simulink model "LimberoGrieel_Robot_Control"  (R2022a)
settings: Solver=VariableStepAuto  StartTime=0.0  StopTime=10.0  RelTol=1e-3
values from neighbouring files (symbols this model uses):
  a = annotation('textbox',dim,'String',str,'FontSize', 20, 'FitBoxToText','on', 'Interpreter', 'tex')    [Experiment_Plot_csv.m]    (also in GRIEEL_transform.m; Gazebo_Plot_csv.m; Grasshopper_Manipulability.m = [a_1; a_2; a_3]; Hexapod_Manipulability_Develop_limits.m = [0, a2, a3])
  alpha = [alpha; alpha; alpha]    [Grasshopper_Manipulability.m]    (also in Hexapod_Manipulability_Develop_limits.m = [-pi/2, 0, 0]; LimberoGrieel_Leg_DH_Modeling_Control.m = [-pi/2,0,0,-pi/2,pi/2, -pi/2, 0]; NewLimbManipulabilityTest.m = [-pi/2, 0, 0]; NewRobot_Manipulability_Develop.m = [-pi/2, 0, 0])
  d = [d; d; d; d]    [Grasshopper_Manipulability.m]    (also in Hexapod_Manipulability_Develop_limits.m = [0, 0, 0]; LimberoGrieel_Leg_DH_Modeling_Control.m = [0,0,0,0,d5,0,d7]; NewLimbManipulabilityTest.m = [d1, 0, 0]; NewRobot_Manipulability_Develop.m = [0,0,0])
  kpp = w_cp    (= 10)    [LimberoGrieel_Leg_DH_Modeling_Control.m]    (also in limberoGrieel_leg_DH.m = 20; limbero_controller.mat; limbero_grieel_dh.m = 20)
  kpv = zeros(1,7)    [LimberoGrieel_Leg_DH_Modeling_Control.m]    (also in limberoGrieel_leg_DH.m; limbero_controller.mat = [361.812023748 321.153278445 225.192840226 266.564703352 222; limbero_grieel_dh.m)
  masses = zeros(N_link,1)    [LimberoGrieel_Leg_DH_Modeling_Control.m]    (also in limberoGrieel_leg_DH.m; limbero_controller.mat = [0.09109 0.12821 0.061841 0.081999 0.110299813858 0.13265995; limbero_grieel_dh.m)
  offset = [offset; offset; offset]    [Grasshopper_Manipulability.m]    (also in Hexapod_Manipulability_Develop_limits.m = [0, 0, 0]; LimberoGrieel_Leg_DH_Modeling_Control.m = zeros(N_link,1); NewLimbManipulabilityTest.m = [0, 0, 0]; NewRobot_Manipulability_Develop.m = [0, 0, 0])
  q0_contact = {}    [LimberoGrieel_Leg_DH_Modeling_Control.m]    (also in LimberoGrieel_Manipulability_Develop.m = q0; LimberoGrieel_Manipulability_Develop_limits.m = q0_wheel; LimberoGrieel_Manipulability_Develop_mesh.m = q0_wheel; LimberoGrieel_Manipulability_Transform.m = q0_wheel)
  r_cm = zeros(N_link,3)    [LimberoGrieel_Leg_DH_Modeling_Control.m]    (also in limberoGrieel_leg_DH.m; limbero_controller.mat = [-0.015062 -0.09917 -0.09702 -9.53000073933e-12 -0.012686054; limbero_grieel_dh.m)
  ROBOT = Robot_model(W, L, Limb, q0, [1 1 1 1], T_tool)    [Experiment_Plot_csv.m]    (also in Gazebo_Plot_csv.m; Grasshopper_Manipulability.m = Robot_model_general(W, L, Limbs, limbs_place,limbs_angle, q0; Hexapod_Manipulability_Develop_limits.m = Robot_model_general(W, L, Limbs, limbs_place,limbs_angle, q0; LimberoGrieel_Manipulability_Develop.m = Robot_model(W, L, Limb, q0_contact_swing, [1 1 1 1], T_tool))
  T_lpf = 1/(w_lpf*2*pi)    (= 0.0106103295395)    [LimberoGrieel_Leg_DH_Modeling_Control.m]    (also in limberoGrieel_leg_DH.m; limbero_controller.mat; limbero_grieel_dh.m)
  T_vel = 1/(w_vel*2*pi)    (= 0.00318309886184)    [LimberoGrieel_Leg_DH_Modeling_Control.m]    (also in limberoGrieel_leg_DH.m; limbero_controller.mat; limbero_grieel_dh.m)
  Tc = Tiv*0.1    (= 0.0666666666667)    [LimberoGrieel_Leg_DH_Modeling_Control.m]    (also in limberoGrieel_leg_DH.m = 0.0333333333333; limbero_controller.mat; limbero_grieel_dh.m = 0.0333333333333)
  Tiv = Tiv*10    (= 0.666666666667)    [LimberoGrieel_Leg_DH_Modeling_Control.m]    (also in limberoGrieel_leg_DH.m = 0.333333333333; limbero_controller.mat; limbero_grieel_dh.m = 0.333333333333)
libraries: roblocks x12
(part 1 of 2)
settings Model: Creator=ale  LastModifiedBy=ale

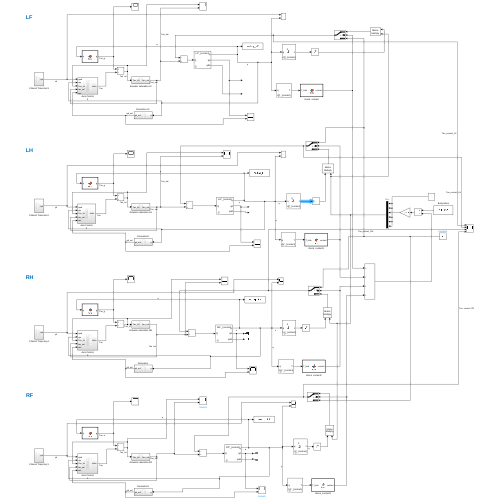
[thumbnail: Simulink's stored preview of the top-level diagram]
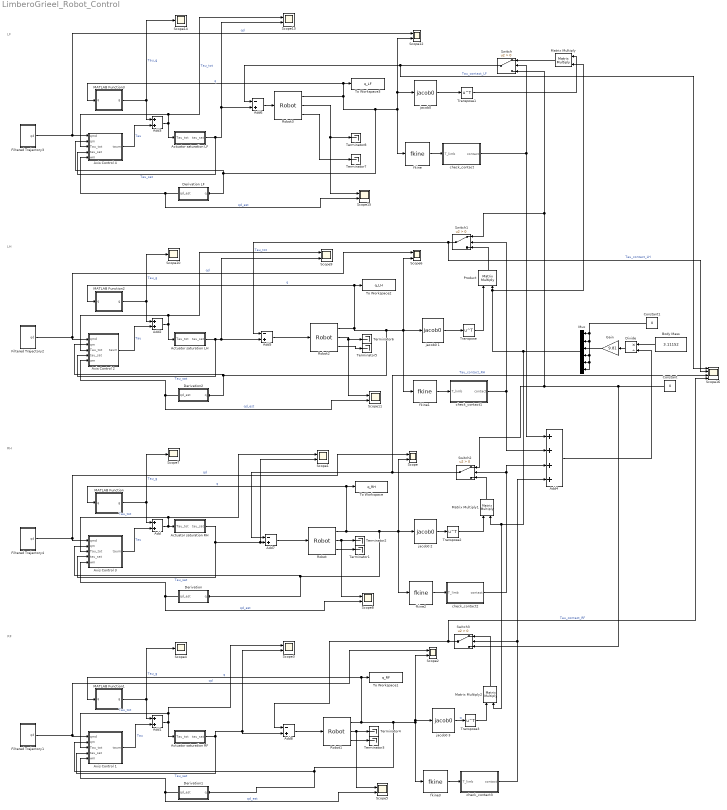
== system LimberoGrieel_Robot_Control ==
  note: RH
  note: RF
  note: LH
  note: LF
  Actuator saturation LF : Subsystem
  Actuator saturation LH : Subsystem
  "Actuator saturation RF " : Subsystem
  Actuator saturation RH : Subsystem
  Add{,1..3} (4 alike) : Sum
  Add4 : Sum  Inputs=++++
  Add{5..8} (4 alike) : Sum  Inputs=-+
  Axis Control 1 : Subsystem
  Axis Control 2 : Subsystem
  Axis Control 3 : Subsystem
  Axis Control 4 : Subsystem
  Body Mass : Constant  Value=3.11152
  Constant : Constant  Value=0
  Constant1 : Constant  Value=0
  Derivation : Subsystem
  Derivation LF : Subsystem
  Derivation1 : Subsystem
  Derivation2 : Subsystem
  Divide : Product  Inputs=*/
  Filtered Trajectory1 : Subsystem
  Filtered Trajectory2 : Subsystem
  Filtered Trajectory3 : Subsystem
  Filtered Trajectory4 : Subsystem
  Gain : Gain  Gain=9.81
  MATLAB Function : MATLAB Function  TreatAsAtomicUnit=on
  MATLAB Function1 : MATLAB Function  TreatAsAtomicUnit=on
  MATLAB Function2 : MATLAB Function  TreatAsAtomicUnit=on
  MATLAB Function3 : MATLAB Function  TreatAsAtomicUnit=on
  Matrix Multiply : Product  Multiplication=Matrix(*)
  Matrix Multiply1 : Product  Multiplication=Matrix(*)
  Matrix Multiply2 : Product  Multiplication=Matrix(*)
  Mux : Mux  Inputs=6
  Product : Product  Multiplication=Matrix(*)
  Robot : roblocks/Arm/Robot  robot=ROBOT(3)  q0=q0_contact(3,:)
  Robot1 : roblocks/Arm/Robot  robot=ROBOT(4)  q0=q0_contact(4,:)
  Robot2 : roblocks/Arm/Robot  robot=ROBOT(2)  q0=q0_contact(2,:)
  Robot3 : roblocks/Arm/Robot  robot=ROBOT(1)  q0=q0_contact(1,:)
  Scope{,1..3,5..6,8..9,11..13,15} (12 alike) : Scope  NumInputPorts=2
  Scope{4,7,10,14} (4 alike) : Scope
  Scope16 : Scope  NumInputPorts=4
  Switch{,1..3} (4 alike) : Switch  Criteria=u2 > Threshold  SaturateOnIntegerOverflow=off  InputSameDT=off
  Terminator{1..8} (8 alike) : Terminator
  To Workspace : ToWorkspace  VariableName=q_RH  SaveFormat=Timeseries  SampleTime=-1
  To Workspace1 : ToWorkspace  VariableName=q_RF  SaveFormat=Timeseries  SampleTime=-1
  To Workspace2 : ToWorkspace  VariableName=q_LH  SaveFormat=Timeseries  SampleTime=-1
  To Workspace3 : ToWorkspace  VariableName=q_LF  SaveFormat=Timeseries  SampleTime=-1
  Transpose{,1..3} (4 alike) : Math  Operator=transpose
  check_contact : MATLAB Function  TreatAsAtomicUnit=on
  check_contact1 : MATLAB Function  TreatAsAtomicUnit=on
  check_contact2 : MATLAB Function  TreatAsAtomicUnit=on
  check_contact3 : MATLAB Function  TreatAsAtomicUnit=on
  fkine : roblocks/Arm/fkine  robot=ROBOT(1)
  fkine1 : roblocks/Arm/fkine  robot=ROBOT(2)
  fkine2 : roblocks/Arm/fkine  robot=ROBOT(3)
  fkine3 : roblocks/Arm/fkine  robot=ROBOT(4)
  "jacob0 " : roblocks/Arm/jacob0   robot=ROBOT(1)
  jacob0 1 : roblocks/Arm/jacob0   robot=ROBOT(2)
  jacob0 2 : roblocks/Arm/jacob0   robot=ROBOT(3)
  jacob0 3 : roblocks/Arm/jacob0   robot=ROBOT(4)
  wires:
  Axis Control 3/1("taum ") -> Add/2  "Tau"
  Robot/3 -> Terminator1/1
  MATLAB Function/1(g) -> Add/1, Scope7/1  "Tau_g"
  Actuator saturation RH/1(tau_sat) -> Scope1/2, Add7/2, Axis Control 3/4(tau_sat)  "Tau_sat"
  Derivation/1(qd_est) -> Scope8/2, Axis Control 3/5(wm)  "qd_est"
  Add/1 -> Axis Control 3/3(Tau_tot), Scope1/1, Actuator saturation RH/1(Tau_tot)  "Tau_tot"
  Filtered Trajectory4/1(qd) -> Axis Control 3/1(qmd), Scope/1  "qd"
  Robot/2 -> Scope8/1, Terminator2/1
  Axis Control 1/1("taum ") -> Add1/2  "Tau"
  Robot1/3 -> Terminator3/1
  MATLAB Function1/1(g) -> Add1/1, Scope4/1  "Tau_g"
  "Actuator saturation RF "/1(tau_sat) -> Axis Control 1/4(tau_sat), Add8/2, Scope3/2  "Tau_sat"
  Derivation1/1(qd_est) -> Scope5/2, Axis Control 1/5(wm)  "qd_est"
  Add1/1 -> Axis Control 1/3(Tau_tot), Scope3/1, "Actuator saturation RF "/1(Tau_tot)  "Tau_tot"
  Filtered Trajectory1/1(qd) -> Axis Control 1/1(qmd), Scope2/1  "qd"
  Robot1/2 -> Scope5/1, Terminator4/1
  Axis Control 2/1("taum ") -> Add2/2  "Tau"
  Robot2/3 -> Terminator5/1
  MATLAB Function2/1(g) -> Add2/1, Scope10/1  "Tau_g"
  Actuator saturation LH/1(tau_sat) -> Axis Control 2/4(tau_sat), Add5/2, Scope9/2  "Tau_sat"
  Derivation2/1(qd_est) -> Scope11/2, Axis Control 2/5(wm)  "qd_est"
  Add2/1 -> Axis Control 2/3(Tau_tot), Scope9/1, Actuator saturation LH/1(Tau_tot)  "Tau_tot"
  Filtered Trajectory2/1(qd) -> Axis Control 2/1(qmd), Scope6/1  "qd"
  Robot2/2 -> Scope11/1, Terminator6/1
  Robot3/1 -> Derivation LF/1(q), Axis Control 4/2(qm), fkine/1, Scope12/2, "jacob0 "/1, MATLAB Function3/1(q), To Workspace3/1  "q"
  Axis Control 4/1("taum ") -> Add3/2  "Tau"
  Robot3/3 -> Terminator7/1
  MATLAB Function3/1(g) -> Add3/1, Scope14/1  "Tau_g"
  Actuator saturation LF/1(tau_sat) -> Axis Control 4/4(tau_sat), Add6/2, Scope13/2  "Tau_sat"
  Derivation LF/1(qd_est) -> Scope15/2, Axis Control 4/5(wm)  "qd_est"
  Add3/1 -> Axis Control 4/3(Tau_tot), Scope13/1, Actuator saturation LF/1(Tau_tot)  "Tau_tot"
  Filtered Trajectory3/1(qd) -> Axis Control 4/1(qmd), Scope12/1  "qd"
  Robot3/2 -> Terminator8/1, Scope15/1
  fkine/1 -> check_contact/1(T_limb)
  Add6/1 -> Robot3/1
  check_contact/1(contact) -> Add4/1, Switch/2
  Robot2/1 -> Derivation2/1(q), Axis Control 2/2(qm), fkine1/1, jacob0 1/1, Scope6/2, MATLAB Function2/1(q), To Workspace2/1  "q"
  check_contact1/1(contact) -> Add4/2, Switch1/2
  fkine1/1 -> check_contact1/1(T_limb)
  Robot/1 -> MATLAB Function/1(q), To Workspace/1, Derivation/1(q), Axis Control 3/2(qm), fkine2/1, jacob0 2/1, Scope/2  "q"
  check_contact2/1(contact) -> Add4/3, Switch2/2
  fkine2/1 -> check_contact2/1(T_limb)
  Robot1/1 -> MATLAB Function1/1(q), To Workspace1/1, Axis Control 1/2(qm), Derivation1/1(q), jacob0 3/1, Scope2/2, fkine3/1  "q"
  check_contact3/1(contact) -> Add4/4, Switch3/2
  fkine3/1 -> check_contact3/1(T_limb)
  Body Mass/1 -> Divide/1
  Add4/1 -> Divide/2
  Divide/1 -> Gain/1
  jacob0 1/1 -> Transpose/1
  Gain/1 -> Mux/3
  Product/1 -> Switch1/3
  Constant/1 -> Switch3/3, Switch1/1, Switch/3, Switch2/1
  Add5/1 -> Robot2/1
  Switch1/1 -> Add5/1, Scope16/2  "Tau_contact_LH"
  Transpose/1 -> Product/1
  "jacob0 "/1 -> Transpose1/1
  Transpose1/1 -> Matrix Multiply/1
  Matrix Multiply/1 -> Switch/1
  Switch/1 -> Scope16/1, Add6/1  "Tau_contact_LF"
  jacob0 2/1 -> Transpose2/1
  Transpose2/1 -> Matrix Multiply1/1
  Matrix Multiply1/1 -> Switch2/3
  Add7/1 -> Robot/1
  Switch2/1 -> Add7/1, Scope16/3  "Tau_contact_RH"
  jacob0 3/1 -> Transpose3/1  "q"
  Transpose3/1 -> Matrix Multiply2/1
  Matrix Multiply2/1 -> Switch3/1
  Add8/1 -> Robot1/1
  Switch3/1 -> Scope16/4, Add8/1  "Tau_contact_RF"
  Constant1/1 -> Mux/6, Mux/5, Mux/4, Mux/2, Mux/1
  Mux/1 -> Matrix Multiply1/2, Matrix Multiply2/2, Matrix Multiply/2, Product/2

== system LimberoGrieel_Robot_Control/Actuator saturation LF ==
  Tau_tot : Inport
  Demux : Demux  Outputs=7
  Mux : Mux  Inputs=7
  Saturation : Saturate  UpperLimit=20.0  LowerLimit=-20.0
  Saturation1 : Saturate  UpperLimit=20.0  LowerLimit=-20.0
  Saturation2 : Saturate  UpperLimit=12.0  LowerLimit=-12.0
  Saturation3 : Saturate  UpperLimit=14.0  LowerLimit=-14.0
  Saturation4 : Saturate  UpperLimit=12.0  LowerLimit=-12.0
  Saturation5 : Saturate  UpperLimit=14.0  LowerLimit=-14.0
  Saturation6 : Saturate  UpperLimit=12.0  LowerLimit=-12.0
  tau_sat : Outport
  wires:
  Saturation6/1 -> Mux/7
  Mux/1 -> tau_sat/1
  Saturation3/1 -> Mux/4
  Tau_tot/1 -> Demux/1
  Demux/4 -> Saturation3/1
  Demux/7 -> Saturation6/1
  Saturation4/1 -> Mux/5
  Saturation1/1 -> Mux/2
  Demux/3 -> Saturation2/1
  Demux/1 -> Saturation/1
  Demux/5 -> Saturation4/1
  Demux/6 -> Saturation5/1
  Demux/2 -> Saturation1/1
  Saturation/1 -> Mux/1
  Saturation5/1 -> Mux/6
  Saturation2/1 -> Mux/3

== system LimberoGrieel_Robot_Control/Actuator saturation LH ==
  Tau_tot : Inport
  Demux : Demux  Outputs=7
  Mux : Mux  Inputs=7
  Saturation : Saturate  UpperLimit=20.0  LowerLimit=-20.0
  Saturation1 : Saturate  UpperLimit=20.0  LowerLimit=-20.0
  Saturation2 : Saturate  UpperLimit=12.0  LowerLimit=-12.0
  Saturation3 : Saturate  UpperLimit=14.0  LowerLimit=-14.0
  Saturation4 : Saturate  UpperLimit=12.0  LowerLimit=-12.0
  Saturation5 : Saturate  UpperLimit=14.0  LowerLimit=-14.0
  Saturation6 : Saturate  UpperLimit=12.0  LowerLimit=-12.0
  tau_sat : Outport
  wires:
  Saturation6/1 -> Mux/7
  Mux/1 -> tau_sat/1
  Saturation3/1 -> Mux/4
  Tau_tot/1 -> Demux/1
  Demux/4 -> Saturation3/1
  Demux/7 -> Saturation6/1
  Saturation4/1 -> Mux/5
  Saturation1/1 -> Mux/2
  Demux/3 -> Saturation2/1
  Demux/1 -> Saturation/1
  Demux/5 -> Saturation4/1
  Demux/6 -> Saturation5/1
  Demux/2 -> Saturation1/1
  Saturation/1 -> Mux/1
  Saturation5/1 -> Mux/6
  Saturation2/1 -> Mux/3

== system LimberoGrieel_Robot_Control/Actuator saturation RF  ==
  Tau_tot : Inport
  Demux : Demux  Outputs=7
  Mux : Mux  Inputs=7
  Saturation : Saturate  UpperLimit=20.0  LowerLimit=-20.0
  Saturation1 : Saturate  UpperLimit=20.0  LowerLimit=-20.0
  Saturation2 : Saturate  UpperLimit=12.0  LowerLimit=-12.0
  Saturation3 : Saturate  UpperLimit=14.0  LowerLimit=-14.0
  Saturation4 : Saturate  UpperLimit=12.0  LowerLimit=-12.0
  Saturation5 : Saturate  UpperLimit=14.0  LowerLimit=-14.0
  Saturation6 : Saturate  UpperLimit=12.0  LowerLimit=-12.0
  tau_sat : Outport
  wires:
  Saturation6/1 -> Mux/7
  Mux/1 -> tau_sat/1
  Saturation3/1 -> Mux/4
  Tau_tot/1 -> Demux/1
  Demux/4 -> Saturation3/1
  Demux/7 -> Saturation6/1
  Saturation4/1 -> Mux/5
  Saturation1/1 -> Mux/2
  Demux/3 -> Saturation2/1
  Demux/1 -> Saturation/1
  Demux/5 -> Saturation4/1
  Demux/6 -> Saturation5/1
  Demux/2 -> Saturation1/1
  Saturation/1 -> Mux/1
  Saturation5/1 -> Mux/6
  Saturation2/1 -> Mux/3

== system LimberoGrieel_Robot_Control/Actuator saturation RH ==
  Tau_tot : Inport
  Demux : Demux  Outputs=7
  Mux : Mux  Inputs=7
  Saturation : Saturate  UpperLimit=20.0  LowerLimit=-20.0
  Saturation1 : Saturate  UpperLimit=20.0  LowerLimit=-20.0
  Saturation2 : Saturate  UpperLimit=12.0  LowerLimit=-12.0
  Saturation3 : Saturate  UpperLimit=14.0  LowerLimit=-14.0
  Saturation4 : Saturate  UpperLimit=12.0  LowerLimit=-12.0
  Saturation5 : Saturate  UpperLimit=14.0  LowerLimit=-14.0
  Saturation6 : Saturate  UpperLimit=12.0  LowerLimit=-12.0
  tau_sat : Outport
  wires:
  Saturation6/1 -> Mux/7
  Mux/1 -> tau_sat/1
  Saturation3/1 -> Mux/4
  Tau_tot/1 -> Demux/1
  Demux/4 -> Saturation3/1
  Demux/7 -> Saturation6/1
  Saturation4/1 -> Mux/5
  Saturation1/1 -> Mux/2
  Demux/3 -> Saturation2/1
  Demux/1 -> Saturation/1
  Demux/5 -> Saturation4/1
  Demux/6 -> Saturation5/1
  Demux/2 -> Saturation1/1
  Saturation/1 -> Mux/1
  Saturation5/1 -> Mux/6
  Saturation2/1 -> Mux/3

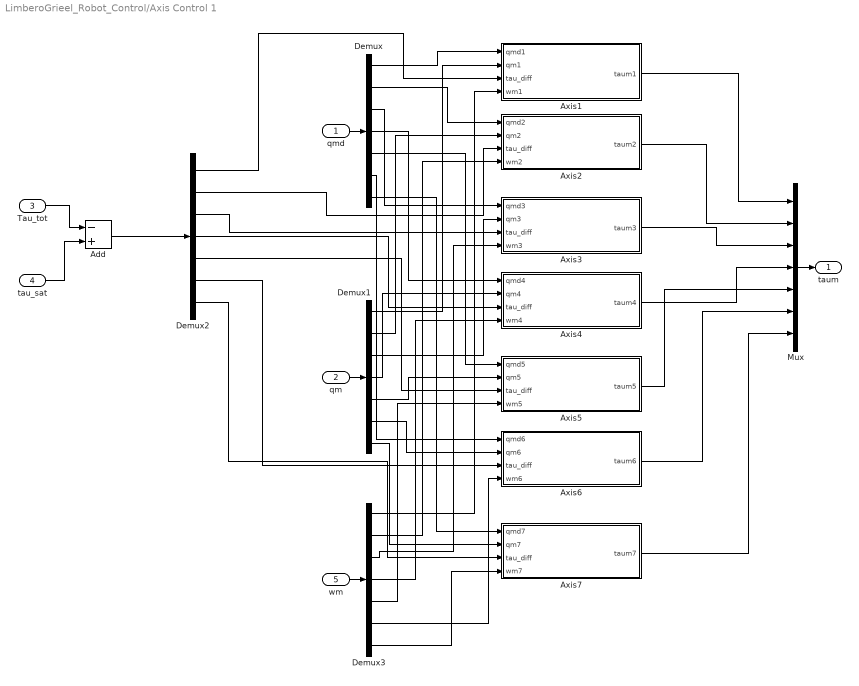
== system LimberoGrieel_Robot_Control/Axis Control 1 ==
  qmd : Inport
  qm : Inport  Port=2
  Tau_tot : Inport  Port=3
  tau_sat : Inport  Port=4
  wm : Inport  Port=5
  Add : Sum  Inputs=-+
  "Axis1 " : Subsystem
  "Axis2 " : Subsystem
  "Axis3 " : Subsystem
  "Axis4 " : Subsystem
  "Axis5 " : Subsystem
  "Axis6 " : Subsystem
  "Axis7 " : Subsystem
  Demux{,1..3} (4 alike) : Demux  Outputs=7
  Mux : Mux  Inputs=7
  "taum " : Outport  VectorParamsAs1DForOutWhenUnconnected=off
  wires:
  "Axis5 "/1(taum5) -> Mux/5
  Demux1/1 -> "Axis1 "/2(qm1)
  "Axis2 "/1(taum2) -> Mux/2
  Demux1/3 -> "Axis3 "/2(qm3)
  Demux/1 -> "Axis1 "/1(qmd1)
  "Axis4 "/1(taum4) -> Mux/4
  "Axis3 "/1(taum3) -> Mux/3
  "Axis6 "/1(taum6) -> Mux/6
  "Axis1 "/1(taum1) -> Mux/1
  Mux/1 -> "taum "/1
  Demux/2 -> "Axis2 "/1(qmd2)
  Demux/4 -> "Axis4 "/1(qmd4)
  Demux/3 -> "Axis3 "/1(qmd3)
  Demux/6 -> "Axis6 "/1(qmd6)
  Demux/5 -> "Axis5 "/1(qmd5)
  Demux1/4 -> "Axis4 "/2(qm4)
  Demux1/6 -> "Axis6 "/2(qm6)
  Demux1/5 -> "Axis5 "/2(qm5)
  Demux1/2 -> "Axis2 "/2(qm2)
  qm/1 -> Demux1/1
  qmd/1 -> Demux/1
  Demux1/7 -> "Axis7 "/2(qm7)
  Demux/7 -> "Axis7 "/1(qmd7)
  "Axis7 "/1(taum7) -> Mux/7
  Tau_tot/1 -> Add/1
  tau_sat/1 -> Add/2
  Demux2/7 -> "Axis7 "/3(tau_diff)
  Add/1 -> Demux2/1
  Demux2/6 -> "Axis6 "/3(tau_diff)
  Demux2/5 -> "Axis5 "/3(tau_diff)
  Demux2/4 -> "Axis4 "/3(tau_diff)
  Demux2/3 -> "Axis3 "/3(tau_diff)
  Demux2/2 -> "Axis2 "/3(tau_diff)
  Demux2/1 -> "Axis1 "/3(tau_diff)
  wm/1 -> Demux3/1
  Demux3/1 -> "Axis1 "/4(wm1)
  Demux3/2 -> "Axis2 "/4(wm2)
  Demux3/3 -> "Axis3 "/4(wm3)
  Demux3/4 -> "Axis4 "/4(wm4)
  Demux3/5 -> "Axis5 "/4(wm5)
  Demux3/6 -> "Axis6 "/4(wm6)
  Demux3/7 -> "Axis7 "/4(wm7)

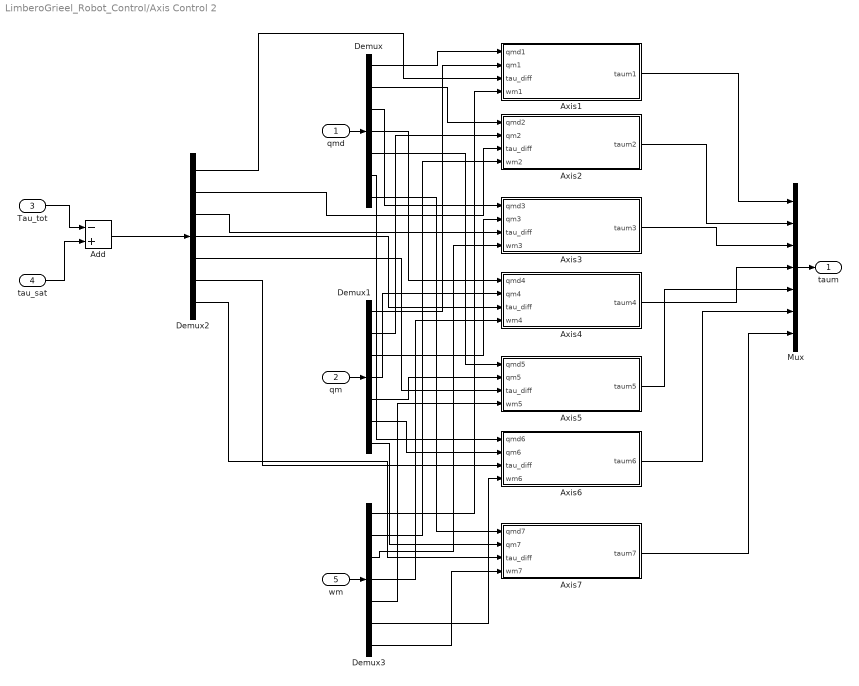
== system LimberoGrieel_Robot_Control/Axis Control 2 ==
  qmd : Inport
  qm : Inport  Port=2
  Tau_tot : Inport  Port=3
  tau_sat : Inport  Port=4
  wm : Inport  Port=5
  Add : Sum  Inputs=-+
  "Axis1 " : Subsystem
  "Axis2 " : Subsystem
  "Axis3 " : Subsystem
  "Axis4 " : Subsystem
  "Axis5 " : Subsystem
  "Axis6 " : Subsystem
  "Axis7 " : Subsystem
  Demux{,1..3} (4 alike) : Demux  Outputs=7
  Mux : Mux  Inputs=7
  "taum " : Outport  VectorParamsAs1DForOutWhenUnconnected=off
  wires:
  "Axis5 "/1(taum5) -> Mux/5
  Demux1/1 -> "Axis1 "/2(qm1)
  "Axis2 "/1(taum2) -> Mux/2
  Demux1/3 -> "Axis3 "/2(qm3)
  Demux/1 -> "Axis1 "/1(qmd1)
  "Axis4 "/1(taum4) -> Mux/4
  "Axis3 "/1(taum3) -> Mux/3
  "Axis6 "/1(taum6) -> Mux/6
  "Axis1 "/1(taum1) -> Mux/1
  Mux/1 -> "taum "/1
  Demux/2 -> "Axis2 "/1(qmd2)
  Demux/4 -> "Axis4 "/1(qmd4)
  Demux/3 -> "Axis3 "/1(qmd3)
  Demux/6 -> "Axis6 "/1(qmd6)
  Demux/5 -> "Axis5 "/1(qmd5)
  Demux1/4 -> "Axis4 "/2(qm4)
  Demux1/6 -> "Axis6 "/2(qm6)
  Demux1/5 -> "Axis5 "/2(qm5)
  Demux1/2 -> "Axis2 "/2(qm2)
  qm/1 -> Demux1/1
  qmd/1 -> Demux/1
  Demux1/7 -> "Axis7 "/2(qm7)
  Demux/7 -> "Axis7 "/1(qmd7)
  "Axis7 "/1(taum7) -> Mux/7
  Tau_tot/1 -> Add/1
  tau_sat/1 -> Add/2
  Demux2/7 -> "Axis7 "/3(tau_diff)
  Add/1 -> Demux2/1
  Demux2/6 -> "Axis6 "/3(tau_diff)
  Demux2/5 -> "Axis5 "/3(tau_diff)
  Demux2/4 -> "Axis4 "/3(tau_diff)
  Demux2/3 -> "Axis3 "/3(tau_diff)
  Demux2/2 -> "Axis2 "/3(tau_diff)
  Demux2/1 -> "Axis1 "/3(tau_diff)
  wm/1 -> Demux3/1
  Demux3/1 -> "Axis1 "/4(wm1)
  Demux3/2 -> "Axis2 "/4(wm2)
  Demux3/3 -> "Axis3 "/4(wm3)
  Demux3/4 -> "Axis4 "/4(wm4)
  Demux3/5 -> "Axis5 "/4(wm5)
  Demux3/6 -> "Axis6 "/4(wm6)
  Demux3/7 -> "Axis7 "/4(wm7)

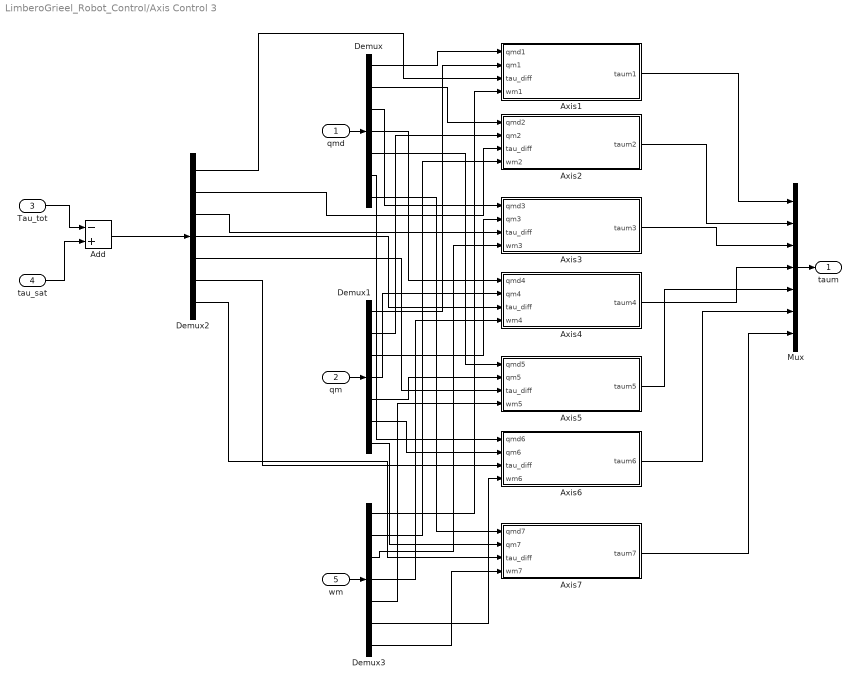
== system LimberoGrieel_Robot_Control/Axis Control 3 ==
  qmd : Inport
  qm : Inport  Port=2
  Tau_tot : Inport  Port=3
  tau_sat : Inport  Port=4
  wm : Inport  Port=5
  Add : Sum  Inputs=-+
  "Axis1 " : Subsystem
  "Axis2 " : Subsystem
  "Axis3 " : Subsystem
  "Axis4 " : Subsystem
  "Axis5 " : Subsystem
  "Axis6 " : Subsystem
  "Axis7 " : Subsystem
  Demux{,1..3} (4 alike) : Demux  Outputs=7
  Mux : Mux  Inputs=7
  "taum " : Outport  VectorParamsAs1DForOutWhenUnconnected=off
  wires:
  "Axis5 "/1(taum5) -> Mux/5
  Demux1/1 -> "Axis1 "/2(qm1)
  "Axis2 "/1(taum2) -> Mux/2
  Demux1/3 -> "Axis3 "/2(qm3)
  Demux/1 -> "Axis1 "/1(qmd1)
  "Axis4 "/1(taum4) -> Mux/4
  "Axis3 "/1(taum3) -> Mux/3
  "Axis6 "/1(taum6) -> Mux/6
  "Axis1 "/1(taum1) -> Mux/1
  Mux/1 -> "taum "/1
  Demux/2 -> "Axis2 "/1(qmd2)
  Demux/4 -> "Axis4 "/1(qmd4)
  Demux/3 -> "Axis3 "/1(qmd3)
  Demux/6 -> "Axis6 "/1(qmd6)
  Demux/5 -> "Axis5 "/1(qmd5)
  Demux1/4 -> "Axis4 "/2(qm4)
  Demux1/6 -> "Axis6 "/2(qm6)
  Demux1/5 -> "Axis5 "/2(qm5)
  Demux1/2 -> "Axis2 "/2(qm2)
  qm/1 -> Demux1/1
  qmd/1 -> Demux/1
  Demux1/7 -> "Axis7 "/2(qm7)
  Demux/7 -> "Axis7 "/1(qmd7)
  "Axis7 "/1(taum7) -> Mux/7
  Tau_tot/1 -> Add/1
  tau_sat/1 -> Add/2
  Demux2/7 -> "Axis7 "/3(tau_diff)
  Add/1 -> Demux2/1
  Demux2/6 -> "Axis6 "/3(tau_diff)
  Demux2/5 -> "Axis5 "/3(tau_diff)
  Demux2/4 -> "Axis4 "/3(tau_diff)
  Demux2/3 -> "Axis3 "/3(tau_diff)
  Demux2/2 -> "Axis2 "/3(tau_diff)
  Demux2/1 -> "Axis1 "/3(tau_diff)
  wm/1 -> Demux3/1
  Demux3/1 -> "Axis1 "/4(wm1)
  Demux3/2 -> "Axis2 "/4(wm2)
  Demux3/3 -> "Axis3 "/4(wm3)
  Demux3/4 -> "Axis4 "/4(wm4)
  Demux3/5 -> "Axis5 "/4(wm5)
  Demux3/6 -> "Axis6 "/4(wm6)
  Demux3/7 -> "Axis7 "/4(wm7)

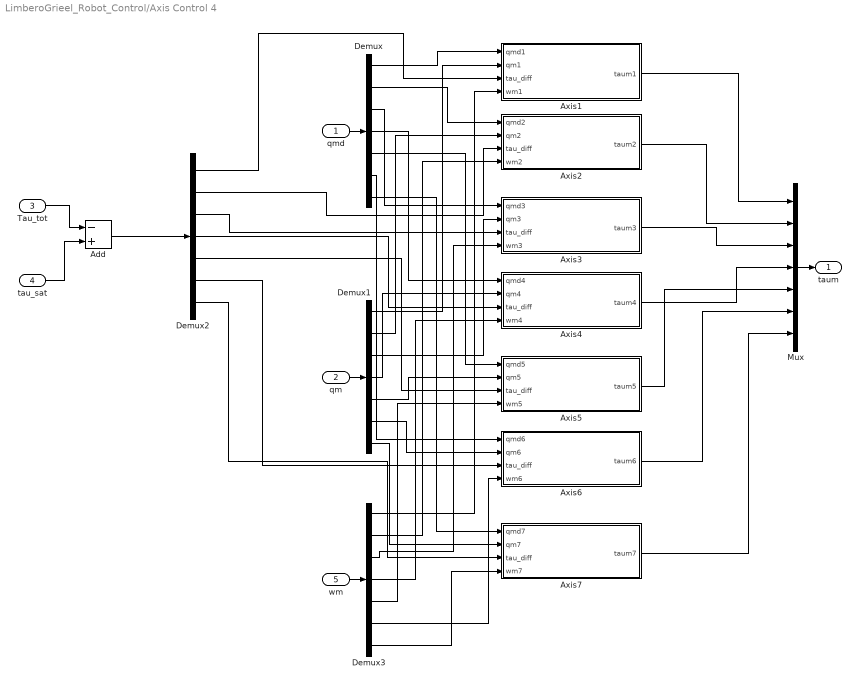
== system LimberoGrieel_Robot_Control/Axis Control 4 ==
  qmd : Inport
  qm : Inport  Port=2
  Tau_tot : Inport  Port=3
  tau_sat : Inport  Port=4
  wm : Inport  Port=5
  Add : Sum  Inputs=-+
  "Axis1 " : Subsystem
  "Axis2 " : Subsystem
  "Axis3 " : Subsystem
  "Axis4 " : Subsystem
  "Axis5 " : Subsystem
  "Axis6 " : Subsystem
  "Axis7 " : Subsystem
  Demux{,1..3} (4 alike) : Demux  Outputs=7
  Mux : Mux  Inputs=7
  "taum " : Outport  VectorParamsAs1DForOutWhenUnconnected=off
  wires:
  "Axis5 "/1(taum5) -> Mux/5
  Demux1/1 -> "Axis1 "/2(qm1)
  "Axis2 "/1(taum2) -> Mux/2
  Demux1/3 -> "Axis3 "/2(qm3)
  Demux/1 -> "Axis1 "/1(qmd1)
  "Axis4 "/1(taum4) -> Mux/4
  "Axis3 "/1(taum3) -> Mux/3
  "Axis6 "/1(taum6) -> Mux/6
  "Axis1 "/1(taum1) -> Mux/1
  Mux/1 -> "taum "/1
  Demux/2 -> "Axis2 "/1(qmd2)
  Demux/4 -> "Axis4 "/1(qmd4)
  Demux/3 -> "Axis3 "/1(qmd3)
  Demux/6 -> "Axis6 "/1(qmd6)
  Demux/5 -> "Axis5 "/1(qmd5)
  Demux1/4 -> "Axis4 "/2(qm4)
  Demux1/6 -> "Axis6 "/2(qm6)
  Demux1/5 -> "Axis5 "/2(qm5)
  Demux1/2 -> "Axis2 "/2(qm2)
  qm/1 -> Demux1/1
  qmd/1 -> Demux/1
  Demux1/7 -> "Axis7 "/2(qm7)
  Demux/7 -> "Axis7 "/1(qmd7)
  "Axis7 "/1(taum7) -> Mux/7
  Tau_tot/1 -> Add/1
  tau_sat/1 -> Add/2
  Demux2/7 -> "Axis7 "/3(tau_diff)
  Add/1 -> Demux2/1
  Demux2/6 -> "Axis6 "/3(tau_diff)
  Demux2/5 -> "Axis5 "/3(tau_diff)
  Demux2/4 -> "Axis4 "/3(tau_diff)
  Demux2/3 -> "Axis3 "/3(tau_diff)
  Demux2/2 -> "Axis2 "/3(tau_diff)
  Demux2/1 -> "Axis1 "/3(tau_diff)
  wm/1 -> Demux3/1
  Demux3/1 -> "Axis1 "/4(wm1)
  Demux3/2 -> "Axis2 "/4(wm2)
  Demux3/3 -> "Axis3 "/4(wm3)
  Demux3/4 -> "Axis4 "/4(wm4)
  Demux3/5 -> "Axis5 "/4(wm5)
  Demux3/6 -> "Axis6 "/4(wm6)
  Demux3/7 -> "Axis7 "/4(wm7)

== system LimberoGrieel_Robot_Control/Derivation ==
  q : Inport
  Demux : Demux  Outputs=7
  Mux : Mux  Inputs=7
  Transfer Fcn{,1..6} (7 alike) : TransferFcn  Numerator=[1 0]  Denominator=[T_vel 1]
  qd_est : Outport
  wires:
  Mux/1 -> qd_est/1
  q/1 -> Demux/1
  Demux/4 -> Transfer Fcn3/1
  Demux/7 -> Transfer Fcn6/1
  Transfer Fcn1/1 -> Mux/2
  Demux/3 -> Transfer Fcn2/1
  Demux/1 -> Transfer Fcn/1
  Demux/5 -> Transfer Fcn4/1
  Demux/6 -> Transfer Fcn5/1
  Demux/2 -> Transfer Fcn1/1
  Transfer Fcn/1 -> Mux/1
  Transfer Fcn6/1 -> Mux/7
  Transfer Fcn5/1 -> Mux/6
  Transfer Fcn4/1 -> Mux/5
  Transfer Fcn3/1 -> Mux/4
  Transfer Fcn2/1 -> Mux/3

== system LimberoGrieel_Robot_Control/Derivation LF ==
  q : Inport
  Demux : Demux  Outputs=7
  Mux : Mux  Inputs=7
  Transfer Fcn{,1..6} (7 alike) : TransferFcn  Numerator=[1 0]  Denominator=[T_vel 1]
  qd_est : Outport
  wires:
  Mux/1 -> qd_est/1
  q/1 -> Demux/1
  Demux/4 -> Transfer Fcn3/1
  Demux/7 -> Transfer Fcn6/1
  Transfer Fcn1/1 -> Mux/2
  Demux/3 -> Transfer Fcn2/1
  Demux/1 -> Transfer Fcn/1
  Demux/5 -> Transfer Fcn4/1
  Demux/6 -> Transfer Fcn5/1
  Demux/2 -> Transfer Fcn1/1
  Transfer Fcn/1 -> Mux/1
  Transfer Fcn6/1 -> Mux/7
  Transfer Fcn5/1 -> Mux/6
  Transfer Fcn4/1 -> Mux/5
  Transfer Fcn3/1 -> Mux/4
  Transfer Fcn2/1 -> Mux/3

== system LimberoGrieel_Robot_Control/Derivation1 ==
  q : Inport
  Demux : Demux  Outputs=7
  Mux : Mux  Inputs=7
  Transfer Fcn{,1..6} (7 alike) : TransferFcn  Numerator=[1 0]  Denominator=[T_vel 1]
  qd_est : Outport
  wires:
  Mux/1 -> qd_est/1
  q/1 -> Demux/1
  Demux/4 -> Transfer Fcn3/1
  Demux/7 -> Transfer Fcn6/1
  Transfer Fcn1/1 -> Mux/2
  Demux/3 -> Transfer Fcn2/1
  Demux/1 -> Transfer Fcn/1
  Demux/5 -> Transfer Fcn4/1
  Demux/6 -> Transfer Fcn5/1
  Demux/2 -> Transfer Fcn1/1
  Transfer Fcn/1 -> Mux/1
  Transfer Fcn6/1 -> Mux/7
  Transfer Fcn5/1 -> Mux/6
  Transfer Fcn4/1 -> Mux/5
  Transfer Fcn3/1 -> Mux/4
  Transfer Fcn2/1 -> Mux/3

== system LimberoGrieel_Robot_Control/Derivation2 ==
  q : Inport
  Demux : Demux  Outputs=7
  Mux : Mux  Inputs=7
  Transfer Fcn{,1..6} (7 alike) : TransferFcn  Numerator=[1 0]  Denominator=[T_vel 1]
  qd_est : Outport
  wires:
  Mux/1 -> qd_est/1
  q/1 -> Demux/1
  Demux/4 -> Transfer Fcn3/1
  Demux/7 -> Transfer Fcn6/1
  Transfer Fcn1/1 -> Mux/2
  Demux/3 -> Transfer Fcn2/1
  Demux/1 -> Transfer Fcn/1
  Demux/5 -> Transfer Fcn4/1
  Demux/6 -> Transfer Fcn5/1
  Demux/2 -> Transfer Fcn1/1
  Transfer Fcn/1 -> Mux/1
  Transfer Fcn6/1 -> Mux/7
  Transfer Fcn5/1 -> Mux/6
  Transfer Fcn4/1 -> Mux/5
  Transfer Fcn3/1 -> Mux/4
  Transfer Fcn2/1 -> Mux/3

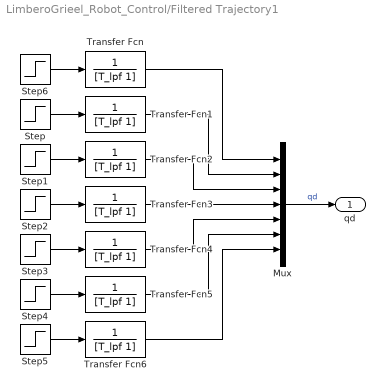
== system LimberoGrieel_Robot_Control/Filtered Trajectory1 ==
  Mux : Mux  Inputs=7
  Step : Step  After=0  SampleTime=0
  Step1 : Step  After=0  SampleTime=0
  Step{2..5} (4 alike) : Step  Time=0  After=0  SampleTime=0
  Step6 : Step  Time=0.5  After=0  SampleTime=0
  Transfer Fcn{,1..6} (7 alike) : TransferFcn  Denominator=[T_lpf 1]
  qd : Outport
  wires:
  Step5/1 -> Transfer Fcn6/1
  Mux/1 -> qd/1  "qd"
  Transfer Fcn1/1 -> Mux/2
  Transfer Fcn4/1 -> Mux/5
  Transfer Fcn2/1 -> Mux/3
  Step6/1 -> Transfer Fcn/1
  Step/1 -> Transfer Fcn1/1
  Step2/1 -> Transfer Fcn3/1
  Transfer Fcn5/1 -> Mux/6
  Transfer Fcn3/1 -> Mux/4
  Transfer Fcn6/1 -> Mux/7
  Transfer Fcn/1 -> Mux/1
  Step4/1 -> Transfer Fcn5/1
  Step1/1 -> Transfer Fcn2/1
  Step3/1 -> Transfer Fcn4/1

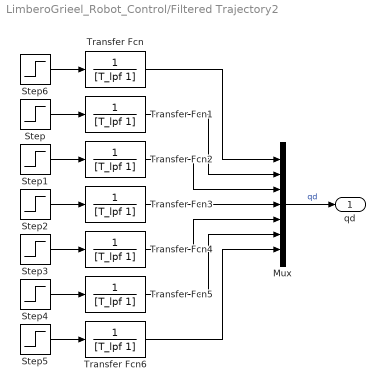
== system LimberoGrieel_Robot_Control/Filtered Trajectory2 ==
  Mux : Mux  Inputs=7
  Step : Step  After=0  SampleTime=0
  Step1 : Step  After=0  SampleTime=0
  Step{2..5} (4 alike) : Step  Time=0  After=0  SampleTime=0
  Step6 : Step  Time=0.5  After=0  SampleTime=0
  Transfer Fcn{,1..6} (7 alike) : TransferFcn  Denominator=[T_lpf 1]
  qd : Outport
  wires:
  Step5/1 -> Transfer Fcn6/1
  Mux/1 -> qd/1  "qd"
  Transfer Fcn1/1 -> Mux/2
  Transfer Fcn4/1 -> Mux/5
  Transfer Fcn2/1 -> Mux/3
  Step6/1 -> Transfer Fcn/1
  Step/1 -> Transfer Fcn1/1
  Step2/1 -> Transfer Fcn3/1
  Transfer Fcn5/1 -> Mux/6
  Transfer Fcn3/1 -> Mux/4
  Transfer Fcn6/1 -> Mux/7
  Transfer Fcn/1 -> Mux/1
  Step4/1 -> Transfer Fcn5/1
  Step1/1 -> Transfer Fcn2/1
  Step3/1 -> Transfer Fcn4/1

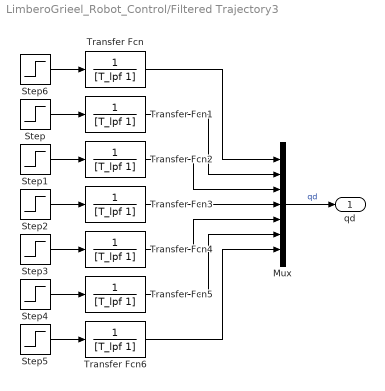
== system LimberoGrieel_Robot_Control/Filtered Trajectory3 ==
  Mux : Mux  Inputs=7
  Step : Step  After=-pi/5  SampleTime=0
  Step1 : Step  After=pi/6  SampleTime=0
  Step{2..5} (4 alike) : Step  Time=0  After=0  SampleTime=0
  Step6 : Step  Time=0.5  After=0  SampleTime=0
  Transfer Fcn{,1..6} (7 alike) : TransferFcn  Denominator=[T_lpf 1]
  qd : Outport
  wires:
  Step5/1 -> Transfer Fcn6/1
  Mux/1 -> qd/1  "qd"
  Transfer Fcn1/1 -> Mux/2
  Transfer Fcn4/1 -> Mux/5
  Transfer Fcn2/1 -> Mux/3
  Step6/1 -> Transfer Fcn/1
  Step/1 -> Transfer Fcn1/1
  Step2/1 -> Transfer Fcn3/1
  Transfer Fcn5/1 -> Mux/6
  Transfer Fcn3/1 -> Mux/4
  Transfer Fcn6/1 -> Mux/7
  Transfer Fcn/1 -> Mux/1
  Step4/1 -> Transfer Fcn5/1
  Step1/1 -> Transfer Fcn2/1
  Step3/1 -> Transfer Fcn4/1

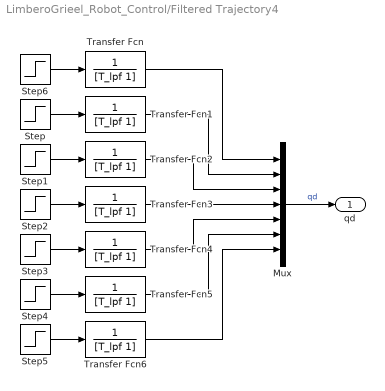
== system LimberoGrieel_Robot_Control/Filtered Trajectory4 ==
  Mux : Mux  Inputs=7
  Step : Step  After=0  SampleTime=0
  Step1 : Step  After=0  SampleTime=0
  Step{2..5} (4 alike) : Step  Time=0  After=0  SampleTime=0
  Step6 : Step  Time=0.5  After=0  SampleTime=0
  Transfer Fcn{,1..6} (7 alike) : TransferFcn  Denominator=[T_lpf 1]
  qd : Outport
  wires:
  Step5/1 -> Transfer Fcn6/1
  Mux/1 -> qd/1  "qd"
  Transfer Fcn1/1 -> Mux/2
  Transfer Fcn4/1 -> Mux/5
  Transfer Fcn2/1 -> Mux/3
  Step6/1 -> Transfer Fcn/1
  Step/1 -> Transfer Fcn1/1
  Step2/1 -> Transfer Fcn3/1
  Transfer Fcn5/1 -> Mux/6
  Transfer Fcn3/1 -> Mux/4
  Transfer Fcn6/1 -> Mux/7
  Transfer Fcn/1 -> Mux/1
  Step4/1 -> Transfer Fcn5/1
  Step1/1 -> Transfer Fcn2/1
  Step3/1 -> Transfer Fcn4/1

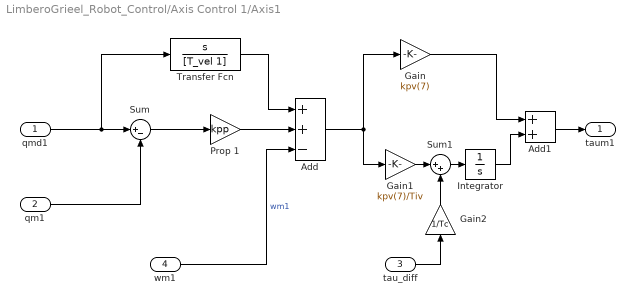
== system LimberoGrieel_Robot_Control/Axis Control 1/Axis1  ==
  qmd1 : Inport
  qm1 : Inport  Port=2
  tau_diff : Inport  Port=3
  wm1 : Inport  Port=4
  Add : Sum  Inputs=++-
  Add1 : Sum
  Gain : Gain  Gain=kpv(7)
  Gain1 : Gain  Gain=kpv(7)/Tiv
  Gain2 : Gain  Gain=1/Tc
  Integrator : Integrator
  Prop 1 : Gain  Gain=kpp
  Sum : Sum  Inputs=|+-
  Sum1 : Sum  Inputs=|++
  Transfer Fcn : TransferFcn  Numerator=[1 0]  Denominator=[T_vel 1]
  taum1 : Outport  VectorParamsAs1DForOutWhenUnconnected=off
  wires:
  Transfer Fcn/1 -> Add/1
  Sum/1 -> Prop 1/1
  qm1/1 -> Sum/2
  Prop 1/1 -> Add/2
  Add/1 -> Gain1/1, Gain/1
  qmd1/1 -> Transfer Fcn/1, Sum/1
  Add1/1 -> taum1/1
  Gain/1 -> Add1/1
  Gain1/1 -> Sum1/1
  Sum1/1 -> Integrator/1
  Integrator/1 -> Add1/2
  Gain2/1 -> Sum1/2
  tau_diff/1 -> Gain2/1
  wm1/1 -> Add/3  "wm1"

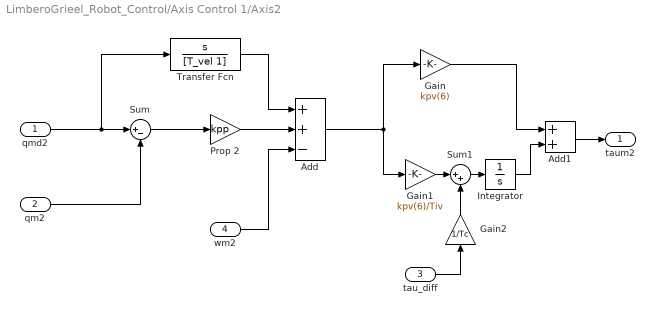
== system LimberoGrieel_Robot_Control/Axis Control 1/Axis2  ==
  qmd2 : Inport
  qm2 : Inport  Port=2
  tau_diff : Inport  Port=3
  wm2 : Inport  Port=4
  Add : Sum  Inputs=++-
  Add1 : Sum
  Gain : Gain  Gain=kpv(6)
  Gain1 : Gain  Gain=kpv(6)/Tiv
  Gain2 : Gain  Gain=1/Tc
  Integrator : Integrator
  Prop 2 : Gain  Gain=kpp
  Sum : Sum  Inputs=|+-
  Sum1 : Sum  Inputs=|++
  Transfer Fcn : TransferFcn  Numerator=[1 0]  Denominator=[T_vel 1]
  taum2 : Outport  VectorParamsAs1DForOutWhenUnconnected=off
  wires:
  Transfer Fcn/1 -> Add/1
  Sum/1 -> Prop 2/1
  qm2/1 -> Sum/2
  Prop 2/1 -> Add/2
  qmd2/1 -> Transfer Fcn/1, Sum/1
  Sum1/1 -> Integrator/1
  Gain1/1 -> Sum1/1
  Gain/1 -> Add1/1
  Add/1 -> Gain1/1, Gain/1
  tau_diff/1 -> Gain2/1
  Integrator/1 -> Add1/2
  Add1/1 -> taum2/1
  Gain2/1 -> Sum1/2
  wm2/1 -> Add/3

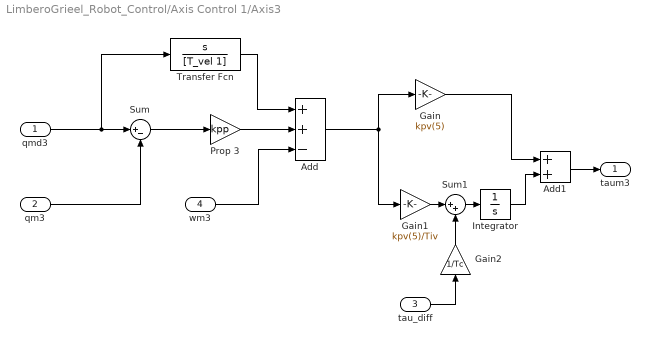
== system LimberoGrieel_Robot_Control/Axis Control 1/Axis3  ==
  qmd3 : Inport
  qm3 : Inport  Port=2
  tau_diff : Inport  Port=3
  wm3 : Inport  Port=4
  Add : Sum  Inputs=++-
  Add1 : Sum
  Gain : Gain  Gain=kpv(5)
  Gain1 : Gain  Gain=kpv(5)/Tiv
  Gain2 : Gain  Gain=1/Tc
  Integrator : Integrator
  Prop 3 : Gain  Gain=kpp
  Sum : Sum  Inputs=|+-
  Sum1 : Sum  Inputs=|++
  Transfer Fcn : TransferFcn  Numerator=[1 0]  Denominator=[T_vel 1]
  taum3 : Outport  VectorParamsAs1DForOutWhenUnconnected=off
  wires:
  Transfer Fcn/1 -> Add/1
  wm3/1 -> Add/3
  Sum/1 -> Prop 3/1
  qm3/1 -> Sum/2
  Prop 3/1 -> Add/2
  qmd3/1 -> Transfer Fcn/1, Sum/1
  Sum1/1 -> Integrator/1
  Gain1/1 -> Sum1/1
  Gain/1 -> Add1/1
  Add/1 -> Gain1/1, Gain/1
  tau_diff/1 -> Gain2/1
  Integrator/1 -> Add1/2
  Add1/1 -> taum3/1
  Gain2/1 -> Sum1/2

== system LimberoGrieel_Robot_Control/Axis Control 1/Axis4  ==
  qmd4 : Inport
  qm4 : Inport  Port=2
  tau_diff : Inport  Port=3
  wm4 : Inport  Port=4
  Add : Sum  Inputs=++-
  Add1 : Sum
  Gain : Gain  Gain=kpv(4)
  Gain1 : Gain  Gain=kpv(4)/Tiv
  Gain2 : Gain  Gain=1/Tc
  Integrator : Integrator
  Prop 4 : Gain  Gain=kpp
  Sum : Sum  Inputs=|+-
  Sum1 : Sum  Inputs=|++
  Transfer Fcn : TransferFcn  Numerator=[1 0]  Denominator=[T_vel 1]
  taum4 : Outport  VectorParamsAs1DForOutWhenUnconnected=off
  wires:
  Transfer Fcn/1 -> Add/1
  wm4/1 -> Add/3
  Sum/1 -> Prop 4/1
  qm4/1 -> Sum/2
  Prop 4/1 -> Add/2
  qmd4/1 -> Transfer Fcn/1, Sum/1
  Sum1/1 -> Integrator/1
  Gain1/1 -> Sum1/1
  Gain/1 -> Add1/1
  Add/1 -> Gain1/1, Gain/1
  tau_diff/1 -> Gain2/1
  Integrator/1 -> Add1/2
  Add1/1 -> taum4/1
  Gain2/1 -> Sum1/2

== system LimberoGrieel_Robot_Control/Axis Control 1/Axis5  ==
  qmd5 : Inport
  qm5 : Inport  Port=2
  tau_diff : Inport  Port=3
  wm5 : Inport  Port=4
  Add : Sum  Inputs=++-
  Add1 : Sum
  Gain : Gain  Gain=kpv(3)
  Gain1 : Gain  Gain=kpv(3)/Tiv
  Gain2 : Gain  Gain=1/Tc
  Integrator : Integrator
  Prop 5 : Gain  Gain=kpp
  Sum : Sum  Inputs=|+-
  Sum1 : Sum  Inputs=|++
  Transfer Fcn : TransferFcn  Numerator=[1 0]  Denominator=[T_vel 1]
  taum5 : Outport  VectorParamsAs1DForOutWhenUnconnected=off
  wires:
  Transfer Fcn/1 -> Add/1
  wm5/1 -> Add/3
  Sum/1 -> Prop 5/1
  qm5/1 -> Sum/2
  Prop 5/1 -> Add/2
  qmd5/1 -> Transfer Fcn/1, Sum/1
  Sum1/1 -> Integrator/1
  Gain1/1 -> Sum1/1
  Gain/1 -> Add1/1
  Add/1 -> Gain1/1, Gain/1
  tau_diff/1 -> Gain2/1
  Integrator/1 -> Add1/2
  Add1/1 -> taum5/1
  Gain2/1 -> Sum1/2

== system LimberoGrieel_Robot_Control/Axis Control 1/Axis6  ==
  qmd6 : Inport
  qm6 : Inport  Port=2
  tau_diff : Inport  Port=3
  wm6 : Inport  Port=4
  Add : Sum  Inputs=++-
  Add1 : Sum
  Gain : Gain  Gain=kpv(2)
  Gain1 : Gain  Gain=kpv(2)/Tiv
  Gain2 : Gain  Gain=1/Tc
  Integrator : Integrator
  Prop 6 : Gain  Gain=kpp
  Sum : Sum  Inputs=|+-
  Sum1 : Sum  Inputs=|++
  Transfer Fcn : TransferFcn  Numerator=[1 0]  Denominator=[T_vel 1]
  taum6 : Outport  VectorParamsAs1DForOutWhenUnconnected=off
  wires:
  Transfer Fcn/1 -> Add/1
  wm6/1 -> Add/3
  Sum/1 -> Prop 6/1
  qm6/1 -> Sum/2
  Prop 6/1 -> Add/2
  qmd6/1 -> Transfer Fcn/1, Sum/1
  Sum1/1 -> Integrator/1
  Gain1/1 -> Sum1/1
  Gain/1 -> Add1/1
  Add/1 -> Gain1/1, Gain/1
  tau_diff/1 -> Gain2/1
  Integrator/1 -> Add1/2
  Add1/1 -> taum6/1
  Gain2/1 -> Sum1/2

== system LimberoGrieel_Robot_Control/Axis Control 1/Axis7  ==
  qmd7 : Inport
  qm7 : Inport  Port=2
  tau_diff : Inport  Port=3
  wm7 : Inport  Port=4
  Add : Sum  Inputs=++-
  Add1 : Sum
  Gain : Gain  Gain=kpv(1)
  Gain1 : Gain  Gain=kpv(1)/Tiv
  Gain2 : Gain  Gain=1/Tc
  Integrator : Integrator
  Prop 7 : Gain  Gain=kpp
  Sum : Sum  Inputs=|+-
  Sum1 : Sum  Inputs=|++
  Transfer Fcn : TransferFcn  Numerator=[1 0]  Denominator=[T_vel 1]
  taum7 : Outport  VectorParamsAs1DForOutWhenUnconnected=off
  wires:
  qmd7/1 -> Transfer Fcn/1, Sum/1
  Prop 7/1 -> Add/2
  qm7/1 -> Sum/2
  Sum/1 -> Prop 7/1
  wm7/1 -> Add/3
  Transfer Fcn/1 -> Add/1
  Sum1/1 -> Integrator/1
  Gain1/1 -> Sum1/1
  Gain/1 -> Add1/1
  Add/1 -> Gain1/1, Gain/1
  tau_diff/1 -> Gain2/1
  Integrator/1 -> Add1/2
  Add1/1 -> taum7/1
  Gain2/1 -> Sum1/2

== system LimberoGrieel_Robot_Control/Axis Control 2/Axis1  ==
  qmd1 : Inport
  qm1 : Inport  Port=2
  tau_diff : Inport  Port=3
  wm1 : Inport  Port=4
  Add : Sum  Inputs=++-
  Add1 : Sum
  Gain : Gain  Gain=kpv(7)
  Gain1 : Gain  Gain=kpv(7)/Tiv
  Gain2 : Gain  Gain=1/Tc
  Integrator : Integrator
  Prop 1 : Gain  Gain=kpp
  Sum : Sum  Inputs=|+-
  Sum1 : Sum  Inputs=|++
  Transfer Fcn : TransferFcn  Numerator=[1 0]  Denominator=[T_vel 1]
  taum1 : Outport  VectorParamsAs1DForOutWhenUnconnected=off
  wires:
  Transfer Fcn/1 -> Add/1
  Sum/1 -> Prop 1/1
  qm1/1 -> Sum/2
  Prop 1/1 -> Add/2
  Add/1 -> Gain1/1, Gain/1
  qmd1/1 -> Transfer Fcn/1, Sum/1
  Add1/1 -> taum1/1
  Gain/1 -> Add1/1
  Gain1/1 -> Sum1/1
  Sum1/1 -> Integrator/1
  Integrator/1 -> Add1/2
  Gain2/1 -> Sum1/2
  tau_diff/1 -> Gain2/1
  wm1/1 -> Add/3  "wm1"

== system LimberoGrieel_Robot_Control/Axis Control 2/Axis2  ==
  qmd2 : Inport
  qm2 : Inport  Port=2
  tau_diff : Inport  Port=3
  wm2 : Inport  Port=4
  Add : Sum  Inputs=++-
  Add1 : Sum
  Gain : Gain  Gain=kpv(6)
  Gain1 : Gain  Gain=kpv(6)/Tiv
  Gain2 : Gain  Gain=1/Tc
  Integrator : Integrator
  Prop 2 : Gain  Gain=kpp
  Sum : Sum  Inputs=|+-
  Sum1 : Sum  Inputs=|++
  Transfer Fcn : TransferFcn  Numerator=[1 0]  Denominator=[T_vel 1]
  taum2 : Outport  VectorParamsAs1DForOutWhenUnconnected=off
  wires:
  Transfer Fcn/1 -> Add/1
  Sum/1 -> Prop 2/1
  qm2/1 -> Sum/2
  Prop 2/1 -> Add/2
  qmd2/1 -> Transfer Fcn/1, Sum/1
  Sum1/1 -> Integrator/1
  Gain1/1 -> Sum1/1
  Gain/1 -> Add1/1
  Add/1 -> Gain1/1, Gain/1
  tau_diff/1 -> Gain2/1
  Integrator/1 -> Add1/2
  Add1/1 -> taum2/1
  Gain2/1 -> Sum1/2
  wm2/1 -> Add/3

== system LimberoGrieel_Robot_Control/Axis Control 2/Axis3  ==
  qmd3 : Inport
  qm3 : Inport  Port=2
  tau_diff : Inport  Port=3
  wm3 : Inport  Port=4
  Add : Sum  Inputs=++-
  Add1 : Sum
  Gain : Gain  Gain=kpv(5)
  Gain1 : Gain  Gain=kpv(5)/Tiv
  Gain2 : Gain  Gain=1/Tc
  Integrator : Integrator
  Prop 3 : Gain  Gain=kpp
  Sum : Sum  Inputs=|+-
  Sum1 : Sum  Inputs=|++
  Transfer Fcn : TransferFcn  Numerator=[1 0]  Denominator=[T_vel 1]
  taum3 : Outport  VectorParamsAs1DForOutWhenUnconnected=off
  wires:
  Transfer Fcn/1 -> Add/1
  wm3/1 -> Add/3
  Sum/1 -> Prop 3/1
  qm3/1 -> Sum/2
  Prop 3/1 -> Add/2
  qmd3/1 -> Transfer Fcn/1, Sum/1
  Sum1/1 -> Integrator/1
  Gain1/1 -> Sum1/1
  Gain/1 -> Add1/1
  Add/1 -> Gain1/1, Gain/1
  tau_diff/1 -> Gain2/1
  Integrator/1 -> Add1/2
  Add1/1 -> taum3/1
  Gain2/1 -> Sum1/2

== system LimberoGrieel_Robot_Control/Axis Control 2/Axis4  ==
  qmd4 : Inport
  qm4 : Inport  Port=2
  tau_diff : Inport  Port=3
  wm4 : Inport  Port=4
  Add : Sum  Inputs=++-
  Add1 : Sum
  Gain : Gain  Gain=kpv(4)
  Gain1 : Gain  Gain=kpv(4)/Tiv
  Gain2 : Gain  Gain=1/Tc
  Integrator : Integrator
  Prop 4 : Gain  Gain=kpp
  Sum : Sum  Inputs=|+-
  Sum1 : Sum  Inputs=|++
  Transfer Fcn : TransferFcn  Numerator=[1 0]  Denominator=[T_vel 1]
  taum4 : Outport  VectorParamsAs1DForOutWhenUnconnected=off
  wires:
  Transfer Fcn/1 -> Add/1
  wm4/1 -> Add/3
  Sum/1 -> Prop 4/1
  qm4/1 -> Sum/2
  Prop 4/1 -> Add/2
  qmd4/1 -> Transfer Fcn/1, Sum/1
  Sum1/1 -> Integrator/1
  Gain1/1 -> Sum1/1
  Gain/1 -> Add1/1
  Add/1 -> Gain1/1, Gain/1
  tau_diff/1 -> Gain2/1
  Integrator/1 -> Add1/2
  Add1/1 -> taum4/1
  Gain2/1 -> Sum1/2

== system LimberoGrieel_Robot_Control/Axis Control 2/Axis5  ==
  qmd5 : Inport
  qm5 : Inport  Port=2
  tau_diff : Inport  Port=3
  wm5 : Inport  Port=4
  Add : Sum  Inputs=++-
  Add1 : Sum
  Gain : Gain  Gain=kpv(3)
  Gain1 : Gain  Gain=kpv(3)/Tiv
  Gain2 : Gain  Gain=1/Tc
  Integrator : Integrator
  Prop 5 : Gain  Gain=kpp
  Sum : Sum  Inputs=|+-
  Sum1 : Sum  Inputs=|++
  Transfer Fcn : TransferFcn  Numerator=[1 0]  Denominator=[T_vel 1]
  taum5 : Outport  VectorParamsAs1DForOutWhenUnconnected=off
  wires:
  Transfer Fcn/1 -> Add/1
  wm5/1 -> Add/3
  Sum/1 -> Prop 5/1
  qm5/1 -> Sum/2
  Prop 5/1 -> Add/2
  qmd5/1 -> Transfer Fcn/1, Sum/1
  Sum1/1 -> Integrator/1
  Gain1/1 -> Sum1/1
  Gain/1 -> Add1/1
  Add/1 -> Gain1/1, Gain/1
  tau_diff/1 -> Gain2/1
  Integrator/1 -> Add1/2
  Add1/1 -> taum5/1
  Gain2/1 -> Sum1/2

== system LimberoGrieel_Robot_Control/Axis Control 2/Axis6  ==
  qmd6 : Inport
  qm6 : Inport  Port=2
  tau_diff : Inport  Port=3
  wm6 : Inport  Port=4
  Add : Sum  Inputs=++-
  Add1 : Sum
  Gain : Gain  Gain=kpv(2)
  Gain1 : Gain  Gain=kpv(2)/Tiv
  Gain2 : Gain  Gain=1/Tc
  Integrator : Integrator
  Prop 6 : Gain  Gain=kpp
  Sum : Sum  Inputs=|+-
  Sum1 : Sum  Inputs=|++
  Transfer Fcn : TransferFcn  Numerator=[1 0]  Denominator=[T_vel 1]
  taum6 : Outport  VectorParamsAs1DForOutWhenUnconnected=off
  wires:
  Transfer Fcn/1 -> Add/1
  wm6/1 -> Add/3
  Sum/1 -> Prop 6/1
  qm6/1 -> Sum/2
  Prop 6/1 -> Add/2
  qmd6/1 -> Transfer Fcn/1, Sum/1
  Sum1/1 -> Integrator/1
  Gain1/1 -> Sum1/1
  Gain/1 -> Add1/1
  Add/1 -> Gain1/1, Gain/1
  tau_diff/1 -> Gain2/1
  Integrator/1 -> Add1/2
  Add1/1 -> taum6/1
  Gain2/1 -> Sum1/2

== system LimberoGrieel_Robot_Control/Axis Control 2/Axis7  ==
  qmd7 : Inport
  qm7 : Inport  Port=2
  tau_diff : Inport  Port=3
  wm7 : Inport  Port=4
  Add : Sum  Inputs=++-
  Add1 : Sum
  Gain : Gain  Gain=kpv(1)
  Gain1 : Gain  Gain=kpv(1)/Tiv
  Gain2 : Gain  Gain=1/Tc
  Integrator : Integrator
  Prop 7 : Gain  Gain=kpp
  Sum : Sum  Inputs=|+-
  Sum1 : Sum  Inputs=|++
  Transfer Fcn : TransferFcn  Numerator=[1 0]  Denominator=[T_vel 1]
  taum7 : Outport  VectorParamsAs1DForOutWhenUnconnected=off
  wires:
  qmd7/1 -> Transfer Fcn/1, Sum/1
  Prop 7/1 -> Add/2
  qm7/1 -> Sum/2
  Sum/1 -> Prop 7/1
  wm7/1 -> Add/3
  Transfer Fcn/1 -> Add/1
  Sum1/1 -> Integrator/1
  Gain1/1 -> Sum1/1
  Gain/1 -> Add1/1
  Add/1 -> Gain1/1, Gain/1
  tau_diff/1 -> Gain2/1
  Integrator/1 -> Add1/2
  Add1/1 -> taum7/1
  Gain2/1 -> Sum1/2

== system LimberoGrieel_Robot_Control/Axis Control 3/Axis1  ==
  qmd1 : Inport
  qm1 : Inport  Port=2
  tau_diff : Inport  Port=3
  wm1 : Inport  Port=4
  Add : Sum  Inputs=++-
  Add1 : Sum
  Gain : Gain  Gain=kpv(7)
  Gain1 : Gain  Gain=kpv(7)/Tiv
  Gain2 : Gain  Gain=1/Tc
  Integrator : Integrator
  Prop 1 : Gain  Gain=kpp
  Sum : Sum  Inputs=|+-
  Sum1 : Sum  Inputs=|++
  Transfer Fcn : TransferFcn  Numerator=[1 0]  Denominator=[T_vel 1]
  taum1 : Outport  VectorParamsAs1DForOutWhenUnconnected=off
  wires:
  Transfer Fcn/1 -> Add/1
  Sum/1 -> Prop 1/1
  qm1/1 -> Sum/2
  Prop 1/1 -> Add/2
  Add/1 -> Gain1/1, Gain/1
  qmd1/1 -> Transfer Fcn/1, Sum/1
  Add1/1 -> taum1/1
  Gain/1 -> Add1/1
  Gain1/1 -> Sum1/1
  Sum1/1 -> Integrator/1
  Integrator/1 -> Add1/2
  Gain2/1 -> Sum1/2
  tau_diff/1 -> Gain2/1
  wm1/1 -> Add/3  "wm1"

== system LimberoGrieel_Robot_Control/Axis Control 3/Axis2  ==
  qmd2 : Inport
  qm2 : Inport  Port=2
  tau_diff : Inport  Port=3
  wm2 : Inport  Port=4
  Add : Sum  Inputs=++-
  Add1 : Sum
  Gain : Gain  Gain=kpv(6)
  Gain1 : Gain  Gain=kpv(6)/Tiv
  Gain2 : Gain  Gain=1/Tc
  Integrator : Integrator
  Prop 2 : Gain  Gain=kpp
  Sum : Sum  Inputs=|+-
  Sum1 : Sum  Inputs=|++
  Transfer Fcn : TransferFcn  Numerator=[1 0]  Denominator=[T_vel 1]
  taum2 : Outport  VectorParamsAs1DForOutWhenUnconnected=off
  wires:
  Transfer Fcn/1 -> Add/1
  Sum/1 -> Prop 2/1
  qm2/1 -> Sum/2
  Prop 2/1 -> Add/2
  qmd2/1 -> Transfer Fcn/1, Sum/1
  Sum1/1 -> Integrator/1
  Gain1/1 -> Sum1/1
  Gain/1 -> Add1/1
  Add/1 -> Gain1/1, Gain/1
  tau_diff/1 -> Gain2/1
  Integrator/1 -> Add1/2
  Add1/1 -> taum2/1
  Gain2/1 -> Sum1/2
  wm2/1 -> Add/3

== system LimberoGrieel_Robot_Control/Axis Control 3/Axis3  ==
  qmd3 : Inport
  qm3 : Inport  Port=2
  tau_diff : Inport  Port=3
  wm3 : Inport  Port=4
  Add : Sum  Inputs=++-
  Add1 : Sum
  Gain : Gain  Gain=kpv(5)
  Gain1 : Gain  Gain=kpv(5)/Tiv
  Gain2 : Gain  Gain=1/Tc
  Integrator : Integrator
  Prop 3 : Gain  Gain=kpp
  Sum : Sum  Inputs=|+-
  Sum1 : Sum  Inputs=|++
  Transfer Fcn : TransferFcn  Numerator=[1 0]  Denominator=[T_vel 1]
  taum3 : Outport  VectorParamsAs1DForOutWhenUnconnected=off
  wires:
  Transfer Fcn/1 -> Add/1
  wm3/1 -> Add/3
  Sum/1 -> Prop 3/1
  qm3/1 -> Sum/2
  Prop 3/1 -> Add/2
  qmd3/1 -> Transfer Fcn/1, Sum/1
  Sum1/1 -> Integrator/1
  Gain1/1 -> Sum1/1
  Gain/1 -> Add1/1
  Add/1 -> Gain1/1, Gain/1
  tau_diff/1 -> Gain2/1
  Integrator/1 -> Add1/2
  Add1/1 -> taum3/1
  Gain2/1 -> Sum1/2

== system LimberoGrieel_Robot_Control/Axis Control 3/Axis4  ==
  qmd4 : Inport
  qm4 : Inport  Port=2
  tau_diff : Inport  Port=3
  wm4 : Inport  Port=4
  Add : Sum  Inputs=++-
  Add1 : Sum
  Gain : Gain  Gain=kpv(4)
  Gain1 : Gain  Gain=kpv(4)/Tiv
  Gain2 : Gain  Gain=1/Tc
  Integrator : Integrator
  Prop 4 : Gain  Gain=kpp
  Sum : Sum  Inputs=|+-
  Sum1 : Sum  Inputs=|++
  Transfer Fcn : TransferFcn  Numerator=[1 0]  Denominator=[T_vel 1]
  taum4 : Outport  VectorParamsAs1DForOutWhenUnconnected=off
  wires:
  Transfer Fcn/1 -> Add/1
  wm4/1 -> Add/3
  Sum/1 -> Prop 4/1
  qm4/1 -> Sum/2
  Prop 4/1 -> Add/2
  qmd4/1 -> Transfer Fcn/1, Sum/1
  Sum1/1 -> Integrator/1
  Gain1/1 -> Sum1/1
  Gain/1 -> Add1/1
  Add/1 -> Gain1/1, Gain/1
  tau_diff/1 -> Gain2/1
  Integrator/1 -> Add1/2
  Add1/1 -> taum4/1
  Gain2/1 -> Sum1/2

== system LimberoGrieel_Robot_Control/Axis Control 3/Axis5  ==
  qmd5 : Inport
  qm5 : Inport  Port=2
  tau_diff : Inport  Port=3
  wm5 : Inport  Port=4
  Add : Sum  Inputs=++-
  Add1 : Sum
  Gain : Gain  Gain=kpv(3)
  Gain1 : Gain  Gain=kpv(3)/Tiv
  Gain2 : Gain  Gain=1/Tc
  Integrator : Integrator
  Prop 5 : Gain  Gain=kpp
  Sum : Sum  Inputs=|+-
  Sum1 : Sum  Inputs=|++
  Transfer Fcn : TransferFcn  Numerator=[1 0]  Denominator=[T_vel 1]
  taum5 : Outport  VectorParamsAs1DForOutWhenUnconnected=off
  wires:
  Transfer Fcn/1 -> Add/1
  wm5/1 -> Add/3
  Sum/1 -> Prop 5/1
  qm5/1 -> Sum/2
  Prop 5/1 -> Add/2
  qmd5/1 -> Transfer Fcn/1, Sum/1
  Sum1/1 -> Integrator/1
  Gain1/1 -> Sum1/1
  Gain/1 -> Add1/1
  Add/1 -> Gain1/1, Gain/1
  tau_diff/1 -> Gain2/1
  Integrator/1 -> Add1/2
  Add1/1 -> taum5/1
  Gain2/1 -> Sum1/2

== system LimberoGrieel_Robot_Control/Axis Control 3/Axis6  ==
  qmd6 : Inport
  qm6 : Inport  Port=2
  tau_diff : Inport  Port=3
  wm6 : Inport  Port=4
  Add : Sum  Inputs=++-
  Add1 : Sum
  Gain : Gain  Gain=kpv(2)
  Gain1 : Gain  Gain=kpv(2)/Tiv
  Gain2 : Gain  Gain=1/Tc
  Integrator : Integrator
  Prop 6 : Gain  Gain=kpp
  Sum : Sum  Inputs=|+-
  Sum1 : Sum  Inputs=|++
  Transfer Fcn : TransferFcn  Numerator=[1 0]  Denominator=[T_vel 1]
  taum6 : Outport  VectorParamsAs1DForOutWhenUnconnected=off
  wires:
  Transfer Fcn/1 -> Add/1
  wm6/1 -> Add/3
  Sum/1 -> Prop 6/1
  qm6/1 -> Sum/2
  Prop 6/1 -> Add/2
  qmd6/1 -> Transfer Fcn/1, Sum/1
  Sum1/1 -> Integrator/1
  Gain1/1 -> Sum1/1
  Gain/1 -> Add1/1
  Add/1 -> Gain1/1, Gain/1
  tau_diff/1 -> Gain2/1
  Integrator/1 -> Add1/2
  Add1/1 -> taum6/1
  Gain2/1 -> Sum1/2

== system LimberoGrieel_Robot_Control/Axis Control 3/Axis7  ==
  qmd7 : Inport
  qm7 : Inport  Port=2
  tau_diff : Inport  Port=3
  wm7 : Inport  Port=4
  Add : Sum  Inputs=++-
  Add1 : Sum
  Gain : Gain  Gain=kpv(1)
  Gain1 : Gain  Gain=kpv(1)/Tiv
  Gain2 : Gain  Gain=1/Tc
  Integrator : Integrator
  Prop 7 : Gain  Gain=kpp
  Sum : Sum  Inputs=|+-
  Sum1 : Sum  Inputs=|++
  Transfer Fcn : TransferFcn  Numerator=[1 0]  Denominator=[T_vel 1]
  taum7 : Outport  VectorParamsAs1DForOutWhenUnconnected=off
  wires:
  qmd7/1 -> Transfer Fcn/1, Sum/1
  Prop 7/1 -> Add/2
  qm7/1 -> Sum/2
  Sum/1 -> Prop 7/1
  wm7/1 -> Add/3
  Transfer Fcn/1 -> Add/1
  Sum1/1 -> Integrator/1
  Gain1/1 -> Sum1/1
  Gain/1 -> Add1/1
  Add/1 -> Gain1/1, Gain/1
  tau_diff/1 -> Gain2/1
  Integrator/1 -> Add1/2
  Add1/1 -> taum7/1
  Gain2/1 -> Sum1/2

== system LimberoGrieel_Robot_Control/Axis Control 4/Axis1  ==
  qmd1 : Inport
  qm1 : Inport  Port=2
  tau_diff : Inport  Port=3
  wm1 : Inport  Port=4
  Add : Sum  Inputs=++-
  Add1 : Sum
  Gain : Gain  Gain=kpv(7)
  Gain1 : Gain  Gain=kpv(7)/Tiv
  Gain2 : Gain  Gain=1/Tc
  Integrator : Integrator
  Prop 1 : Gain  Gain=kpp
  Sum : Sum  Inputs=|+-
  Sum1 : Sum  Inputs=|++
  Transfer Fcn : TransferFcn  Numerator=[1 0]  Denominator=[T_vel 1]
  taum1 : Outport  VectorParamsAs1DForOutWhenUnconnected=off
  wires:
  Transfer Fcn/1 -> Add/1
  Sum/1 -> Prop 1/1
  qm1/1 -> Sum/2
  Prop 1/1 -> Add/2
  Add/1 -> Gain1/1, Gain/1
  qmd1/1 -> Transfer Fcn/1, Sum/1
  Add1/1 -> taum1/1
  Gain/1 -> Add1/1
  Gain1/1 -> Sum1/1
  Sum1/1 -> Integrator/1
  Integrator/1 -> Add1/2
  Gain2/1 -> Sum1/2
  tau_diff/1 -> Gain2/1
  wm1/1 -> Add/3  "wm1"

== system LimberoGrieel_Robot_Control/Axis Control 4/Axis2  ==
  qmd2 : Inport
  qm2 : Inport  Port=2
  tau_diff : Inport  Port=3
  wm2 : Inport  Port=4
  Add : Sum  Inputs=++-
  Add1 : Sum
  Gain : Gain  Gain=kpv(6)
  Gain1 : Gain  Gain=kpv(6)/Tiv
  Gain2 : Gain  Gain=1/Tc
  Integrator : Integrator
  Prop 2 : Gain  Gain=kpp
  Sum : Sum  Inputs=|+-
  Sum1 : Sum  Inputs=|++
  Transfer Fcn : TransferFcn  Numerator=[1 0]  Denominator=[T_vel 1]
  taum2 : Outport  VectorParamsAs1DForOutWhenUnconnected=off
  wires:
  Transfer Fcn/1 -> Add/1
  Sum/1 -> Prop 2/1
  qm2/1 -> Sum/2
  Prop 2/1 -> Add/2
  qmd2/1 -> Transfer Fcn/1, Sum/1
  Sum1/1 -> Integrator/1
  Gain1/1 -> Sum1/1
  Gain/1 -> Add1/1
  Add/1 -> Gain1/1, Gain/1
  tau_diff/1 -> Gain2/1
  Integrator/1 -> Add1/2
  Add1/1 -> taum2/1
  Gain2/1 -> Sum1/2
  wm2/1 -> Add/3

== system LimberoGrieel_Robot_Control/Axis Control 4/Axis3  ==
  qmd3 : Inport
  qm3 : Inport  Port=2
  tau_diff : Inport  Port=3
  wm3 : Inport  Port=4
  Add : Sum  Inputs=++-
  Add1 : Sum
  Gain : Gain  Gain=kpv(5)
  Gain1 : Gain  Gain=kpv(5)/Tiv
  Gain2 : Gain  Gain=1/Tc
  Integrator : Integrator
  Prop 3 : Gain  Gain=kpp
  Sum : Sum  Inputs=|+-
  Sum1 : Sum  Inputs=|++
  Transfer Fcn : TransferFcn  Numerator=[1 0]  Denominator=[T_vel 1]
  taum3 : Outport  VectorParamsAs1DForOutWhenUnconnected=off
  wires:
  Transfer Fcn/1 -> Add/1
  wm3/1 -> Add/3
  Sum/1 -> Prop 3/1
  qm3/1 -> Sum/2
  Prop 3/1 -> Add/2
  qmd3/1 -> Transfer Fcn/1, Sum/1
  Sum1/1 -> Integrator/1
  Gain1/1 -> Sum1/1
  Gain/1 -> Add1/1
  Add/1 -> Gain1/1, Gain/1
  tau_diff/1 -> Gain2/1
  Integrator/1 -> Add1/2
  Add1/1 -> taum3/1
  Gain2/1 -> Sum1/2

== system LimberoGrieel_Robot_Control/Axis Control 4/Axis4  ==
  qmd4 : Inport
  qm4 : Inport  Port=2
  tau_diff : Inport  Port=3
  wm4 : Inport  Port=4
  Add : Sum  Inputs=++-
  Add1 : Sum
  Gain : Gain  Gain=kpv(4)
  Gain1 : Gain  Gain=kpv(4)/Tiv
  Gain2 : Gain  Gain=1/Tc
  Integrator : Integrator
  Prop 4 : Gain  Gain=kpp
  Sum : Sum  Inputs=|+-
  Sum1 : Sum  Inputs=|++
  Transfer Fcn : TransferFcn  Numerator=[1 0]  Denominator=[T_vel 1]
  taum4 : Outport  VectorParamsAs1DForOutWhenUnconnected=off
  wires:
  Transfer Fcn/1 -> Add/1
  wm4/1 -> Add/3
  Sum/1 -> Prop 4/1
  qm4/1 -> Sum/2
  Prop 4/1 -> Add/2
  qmd4/1 -> Transfer Fcn/1, Sum/1
  Sum1/1 -> Integrator/1
  Gain1/1 -> Sum1/1
  Gain/1 -> Add1/1
  Add/1 -> Gain1/1, Gain/1
  tau_diff/1 -> Gain2/1
  Integrator/1 -> Add1/2
  Add1/1 -> taum4/1
  Gain2/1 -> Sum1/2

== system LimberoGrieel_Robot_Control/Axis Control 4/Axis5  ==
  qmd5 : Inport
  qm5 : Inport  Port=2
  tau_diff : Inport  Port=3
  wm5 : Inport  Port=4
  Add : Sum  Inputs=++-
  Add1 : Sum
  Gain : Gain  Gain=kpv(3)
  Gain1 : Gain  Gain=kpv(3)/Tiv
  Gain2 : Gain  Gain=1/Tc
  Integrator : Integrator
  Prop 5 : Gain  Gain=kpp
  Sum : Sum  Inputs=|+-
  Sum1 : Sum  Inputs=|++
  Transfer Fcn : TransferFcn  Numerator=[1 0]  Denominator=[T_vel 1]
  taum5 : Outport  VectorParamsAs1DForOutWhenUnconnected=off
  wires:
  Transfer Fcn/1 -> Add/1
  wm5/1 -> Add/3
  Sum/1 -> Prop 5/1
  qm5/1 -> Sum/2
  Prop 5/1 -> Add/2
  qmd5/1 -> Transfer Fcn/1, Sum/1
  Sum1/1 -> Integrator/1
  Gain1/1 -> Sum1/1
  Gain/1 -> Add1/1
  Add/1 -> Gain1/1, Gain/1
  tau_diff/1 -> Gain2/1
  Integrator/1 -> Add1/2
  Add1/1 -> taum5/1
  Gain2/1 -> Sum1/2

== system LimberoGrieel_Robot_Control/Axis Control 4/Axis6  ==
  qmd6 : Inport
  qm6 : Inport  Port=2
  tau_diff : Inport  Port=3
  wm6 : Inport  Port=4
  Add : Sum  Inputs=++-
  Add1 : Sum
  Gain : Gain  Gain=kpv(2)
  Gain1 : Gain  Gain=kpv(2)/Tiv
  Gain2 : Gain  Gain=1/Tc
  Integrator : Integrator
  Prop 6 : Gain  Gain=kpp
  Sum : Sum  Inputs=|+-
  Sum1 : Sum  Inputs=|++
  Transfer Fcn : TransferFcn  Numerator=[1 0]  Denominator=[T_vel 1]
  taum6 : Outport  VectorParamsAs1DForOutWhenUnconnected=off
  wires:
  Transfer Fcn/1 -> Add/1
  wm6/1 -> Add/3
  Sum/1 -> Prop 6/1
  qm6/1 -> Sum/2
  Prop 6/1 -> Add/2
  qmd6/1 -> Transfer Fcn/1, Sum/1
  Sum1/1 -> Integrator/1
  Gain1/1 -> Sum1/1
  Gain/1 -> Add1/1
  Add/1 -> Gain1/1, Gain/1
  tau_diff/1 -> Gain2/1
  Integrator/1 -> Add1/2
  Add1/1 -> taum6/1
  Gain2/1 -> Sum1/2
